simulink model "sampleModel7126_pp_1_1"  (R2018a)
settings: Solver=VariableStepAuto  StartTime=0.0  StopTime=10.0  RelTol=1e-3
undefined symbols (not defined in the file): DiscIntNeverNeededParam
libraries: simulink x367
(part 11 of 12)

== system sampleModel7126_pp_1_1/cfblk298/cfblk16 ==
  cfblk1 : Inport
  Action Port : ActionPort  ActionType=else
  cfblk10 : Subsystem  TreatAsAtomicUnit=on
  cfblk11 : Delay  ShowEnablePort=on
      settings: InputPortMap=u0,e6
  cfblk12 : simulink/Discrete/Transfer Fcn Lead or Lag  PoleZ=0.95  ZeroZ=0.75  ICPrevOutput=0.0  ICPrevInput=0.0  DoSatur=off
      settings: SourceProductName=Simulink  SourceProductBaseCode=SL
  cfblk13 : simulink/Discrete/Transfer Fcn Real Zero  ZeroZ=0.75  ICPrevInput=0.0  DoSatur=off
      settings: SourceProductName=Simulink  SourceProductBaseCode=SL
  cfblk14 : simulink/Continuous/PID Controller (2DOF)  Controller=PID  TimeDomain=Discrete-time  SampleTime=-1  IntegratorMethod=Forward Euler  FilterMethod=Forward Euler  Form=Parallel  UseFilter=on  ControllerParametersSource=internal  P=1  I=1  D=0  N=100  b=1  c=1  InitialConditionSource=internal  InitialConditionForIntegrator=0  InitialConditionForFilter=0  ExternalReset=none  LimitOutput=off  UpperSaturationLimit=inf  LowerSaturationLimit=-inf  LinearizeAsGain=off  AntiWindupMode=none  Kb=1  TrackingMode=off  Kt=1  PParamMin=[]  PParamMax=[]  IParamMin=[]  IParamMax=[]  DParamMin=[]  DParamMax=[]  NParamMin=[]  NParamMax=[]  bParamMin=[]  bParamMax=[]  cParamMin=[]  cParamMax=[]  KbParamMin=[]  KbParamMax=[]  KtParamMin=[]  KtParamMax=[]  POutMin=[]  POutMax=[]  IOutMin=[]  IOutMax=[]  DOutMin=[]  DOutMax=[]  NOutMin=[]  NOutMax=[]  bOutMin=[]  bOutMax=[]  cOutMin=[]  cOutMax=[]  KbOutMin=[]  KbOutMax=[]  KtOutMin=[]  KtOutMax=[]  IntegratorOutMin=[]  IntegratorOutMax=[]  FilterOutMin=[]  FilterOutMax=[]  SumOutMin=[]  SumOutMax=[]  Sum1OutMin=[]  Sum1OutMax=[]  Sum2OutMin=[]  Sum2OutMax=[]  Sum3OutMin=[]  Sum3OutMax=[]  SumI1OutMin=[]  SumI1OutMax=[]  SumI2OutMin=[]  SumI2OutMax=[]  SumI3OutMin=[]  SumI3OutMax=[]  SumDOutMin=[]  SumDOutMax=[]  SaturationOutMin=[]  SaturationOutMax=[]  IntegratorContinuousStateAttributes=''  IntegratorStateMustResolveToSignalObject=off  IntegratorRTWStateStorageClass=Auto  FilterContinuousStateAttributes=''  FilterStateMustResolveToSignalObject=off  FilterRTWStateStorageClass=Auto  DifferentiatorICPrevScaledInput=0  DifferentiatorOutMin=[]  DifferentiatorOutMax=[]  FilterDiffOutCoefMin=[]  FilterDiffOutCoefMax=[]  SumDenOutMin=[]  SumDenOutMax=[]  SumNumOutMin=[]  SumNumOutMax=[]  ReciprocalOutMin=[]  ReciprocalOutMax=[]  DivideOutMin=[]  DivideOutMax=[]  TunerSelectOption=Transfer Function Based (PID Tuner App)
  cfblk15 : Delay
  cfblk16 : Delay
  cfblk3 : DiscreteFir
  cfblk4 : simulink/Discrete/Tapped Delay  vinit=0.0  samptime=-1  NumDelays=1  DelayOrder=Oldest  includeCurrent=off
  cfblk5 : simulink/Discrete/Transfer Fcn Real Zero  ZeroZ=0.75  ICPrevInput=0.0  DoSatur=off
      settings: SourceProductName=Simulink  SourceProductBaseCode=SL
  cfblk6 : Subsystem  TreatAsAtomicUnit=on
  cfblk7 : simulink/Continuous/PID Controller  Controller=PID  TimeDomain=Discrete-time  SampleTime=-1  IntegratorMethod=Forward Euler  FilterMethod=Forward Euler  Form=Parallel  UseFilter=on  ControllerParametersSource=internal  P=1  I=1  D=0  N=100  InitialConditionSource=internal  InitialConditionForIntegrator=0  InitialConditionForFilter=0  ExternalReset=none  LimitOutput=off  UpperSaturationLimit=inf  LowerSaturationLimit=-inf  LinearizeAsGain=off  AntiWindupMode=none  Kb=1  TrackingMode=off  Kt=1  PParamMin=[]  PParamMax=[]  IParamMin=[]  IParamMax=[]  DParamMin=[]  DParamMax=[]  NParamMin=[]  NParamMax=[]  KbParamMin=[]  KbParamMax=[]  KtParamMin=[]  KtParamMax=[]  POutMin=[]  POutMax=[]  IOutMin=[]  IOutMax=[]  DOutMin=[]  DOutMax=[]  NOutMin=[]  NOutMax=[]  KbOutMin=[]  KbOutMax=[]  KtOutMin=[]  KtOutMax=[]  IntegratorOutMin=[]  IntegratorOutMax=[]  FilterOutMin=[]  FilterOutMax=[]  SumOutMin=[]  SumOutMax=[]  SumI1OutMin=[]  SumI1OutMax=[]  SumI2OutMin=[]  SumI2OutMax=[]  SumI3OutMin=[]  SumI3OutMax=[]  SumDOutMin=[]  SumDOutMax=[]  SaturationOutMin=[]  SaturationOutMax=[]  IntegratorContinuousStateAttributes=''  IntegratorStateMustResolveToSignalObject=off  IntegratorRTWStateStorageClass=Auto  FilterContinuousStateAttributes=''  FilterStateMustResolveToSignalObject=off  FilterRTWStateStorageClass=Auto  DifferentiatorICPrevScaledInput=0  DifferentiatorOutMin=[]  DifferentiatorOutMax=[]  FilterDiffOutCoefMin=[]  FilterDiffOutCoefMax=[]  SumDenOutMin=[]  SumDenOutMax=[]  SumNumOutMin=[]  SumNumOutMax=[]  ReciprocalOutMin=[]  ReciprocalOutMax=[]  DivideOutMin=[]  DivideOutMax=[]  TunerSelectOption=Transfer Function Based (PID Tuner App)
  cfblk8 : Subsystem  TreatAsAtomicUnit=on
  cfblk9 : simulink/Discrete/Transfer Fcn Real Zero  ZeroZ=0.75  ICPrevInput=0.0  DoSatur=off
      settings: SourceProductName=Simulink  SourceProductBaseCode=SL
  cyemi_{1315..1330} (16 alike) : DataTypeConversion  OutDataTypeStr=double
  emi_1449 : Subsystem  TreatAsAtomicUnit=on
  emi_1451 : If  IfExpression=0 <= u1  SampleTime=[1 0]
  emi_1452 : DataTypeConversion  OutDataTypeStr=double
  emi_1815 : Subsystem  TreatAsAtomicUnit=on
  emi_1817 : If  IfExpression=0 <= u1
  emi_1818 : DataTypeConversion  OutDataTypeStr=double
  emi_905 : Subsystem  TreatAsAtomicUnit=on
  emi_907 : If  IfExpression=0 <= u1  SampleTime=[1 0]
  emi_908 : DataTypeConversion  OutDataTypeStr=double
  cfblk2 : Outport
  wires:
  cfblk7/1 -> cyemi_1319/1, cyemi_1325/1
  cfblk9/1 -> cyemi_1322/1, cyemi_1326/1
  cfblk1/1 -> cyemi_1315/1
  cyemi_1316/1 -> cfblk11/1
  cfblk15/1 -> cyemi_1316/1
  cyemi_1317/1 -> cfblk11/2
  cfblk14/1 -> cyemi_1317/1
  cyemi_1318/1 -> cfblk12/1
  cyemi_1319/1 -> cfblk13/1
  cyemi_1320/1 -> cfblk14/1
  cfblk12/1 -> cyemi_1320/1
  cyemi_1321/1 -> cfblk14/2
  cfblk16/1 -> cyemi_1321/1
  cyemi_1322/1 -> cfblk15/1
  cyemi_1323/1 -> cfblk16/1
  cyemi_1324/1 -> cfblk3/1
  cfblk13/1 -> cyemi_1324/1
  cyemi_1325/1 -> cfblk4/1
  cyemi_1326/1 -> cfblk5/1
  cfblk3/1 -> cyemi_1327/1
  cyemi_1328/1 -> cfblk7/1
  cfblk5/1 -> cyemi_1328/1
  cfblk4/1 -> cyemi_1329/1, emi_908/1, emi_1818/1
  cyemi_1330/1 -> cfblk9/1
  cfblk11/1 -> cyemi_1330/1
  cyemi_1327/1 -> cfblk6/1(emi_903)
  cfblk6/1(emi_904) -> cyemi_1323/1
  emi_907/1 -> cfblk6/Action
  emi_907/2 -> emi_905/Action
  emi_908/1 -> emi_907/1
  cyemi_1329/1 -> cfblk8/1(emi_1447)
  cfblk8/1(emi_1448) -> cfblk2/1
  emi_1451/1 -> cfblk8/Action
  emi_1451/2 -> emi_1449/Action
  emi_1452/1 -> emi_1451/1
  cyemi_1315/1 -> cfblk10/1(emi_1813)
  cfblk10/1(emi_1814) -> emi_1452/1, cyemi_1318/1
  emi_1817/1 -> cfblk10/Action
  emi_1817/2 -> emi_1815/Action
  emi_1818/1 -> emi_1817/1

== system sampleModel7126_pp_1_1/cfblk298/cfblk3 ==
  emi_1703 : Inport
  Action Port : ActionPort  ActionType=then
  cfblk3 : Delay
  emi_1704 : Outport
  wires:
  emi_1703/1 -> cfblk3/1
  cfblk3/1 -> emi_1704/1

== system sampleModel7126_pp_1_1/cfblk298/cfblk4 ==
  emi_1291 : Inport
  Action Port : ActionPort  ActionType=then
  cfblk4 : Delay
  emi_1292 : Outport
  wires:
  emi_1291/1 -> cfblk4/1
  cfblk4/1 -> emi_1292/1

== system sampleModel7126_pp_1_1/cfblk298/emi_1293 ==
  Action Port : ActionPort  ActionType=else
  emi_1294 : Assertion

== system sampleModel7126_pp_1_1/cfblk298/emi_1705 ==
  Action Port : ActionPort  ActionType=else
  emi_1706 : Assertion

== system sampleModel7126_pp_1_1/cfblk245/cfblk18/cfblk3 ==
  emi_65 : Inport
  Action Port : ActionPort  ActionType=then
  cfblk3 : UnitDelay  SampleTime=-1
  emi_66 : Outport
  wires:
  emi_65/1 -> cfblk3/1
  cfblk3/1 -> emi_66/1

== system sampleModel7126_pp_1_1/cfblk245/cfblk18/cfblk5 ==
  emi_460 : Inport
  Action Port : ActionPort  ActionType=then
  cfblk5 : DiscreteFilter
  emi_461 : Outport
  wires:
  emi_460/1 -> cfblk5/1
  cfblk5/1 -> emi_461/1

== system sampleModel7126_pp_1_1/cfblk245/cfblk18/cfblk7 ==
  emi_202 : Inport
  Action Port : ActionPort  ActionType=then
  cfblk7 : simulink/Discrete/Transfer Fcn Lead or Lag  PoleZ=0.95  ZeroZ=0.75  ICPrevOutput=0.0  ICPrevInput=0.0  DoSatur=off
      settings: SourceProductName=Simulink  SourceProductBaseCode=SL
  emi_203 : Outport
  wires:
  emi_202/1 -> cfblk7/1
  cfblk7/1 -> emi_203/1

== system sampleModel7126_pp_1_1/cfblk245/cfblk18/cfblk8 ==
  emi_1710 : Inport
  emi_1711 : Inport  Port=2
  Action Port : ActionPort  ActionType=then
  cfblk8 : Delay  DelayLengthSource=Input port
      settings: InputPortMap=u0,p1
  emi_1712 : Outport
  wires:
  emi_1710/1 -> cfblk8/1
  emi_1711/1 -> cfblk8/2
  cfblk8/1 -> emi_1712/1

== system sampleModel7126_pp_1_1/cfblk245/cfblk18/emi_1713 ==
  Action Port : ActionPort  ActionType=else
  emi_1714 : Assertion

== system sampleModel7126_pp_1_1/cfblk245/cfblk18/emi_204 ==
  Action Port : ActionPort  ActionType=else
  emi_205 : Assertion

== system sampleModel7126_pp_1_1/cfblk245/cfblk18/emi_462 ==
  Action Port : ActionPort  ActionType=else
  emi_463 : Assertion

== system sampleModel7126_pp_1_1/cfblk245/cfblk18/emi_67 ==
  Action Port : ActionPort  ActionType=else
  emi_68 : Assertion

== system sampleModel7126_pp_1_1/cfblk245/cfblk19/cfblk13 ==
  emi_1942 : Inport
  Action Port : ActionPort  ActionType=then
  cfblk13 : Delay
  emi_1943 : Outport
  wires:
  emi_1942/1 -> cfblk13/1
  cfblk13/1 -> emi_1943/1

== system sampleModel7126_pp_1_1/cfblk245/cfblk19/cfblk6 ==
  emi_2159 : Inport
  Action Port : ActionPort  ActionType=then
  cfblk6 : simulink/Discrete/Transfer Fcn First Order  PoleZ=0.95  ICPrevOutput=0.0  DoSatur=off
      settings: SourceProductName=Simulink
  emi_2160 : Outport
  wires:
  emi_2159/1 -> cfblk6/1
  cfblk6/1 -> emi_2160/1

== system sampleModel7126_pp_1_1/cfblk245/cfblk19/emi_1944 ==
  Action Port : ActionPort  ActionType=else
  emi_1945 : Assertion

== system sampleModel7126_pp_1_1/cfblk245/cfblk19/emi_2161 ==
  Action Port : ActionPort  ActionType=else
  emi_2162 : Assertion

== system sampleModel7126_pp_1_1/cfblk246/cfblk10/cfblk10 ==
  emi_152 : Inport
  Action Port : ActionPort  ActionType=then
  cfblk10 : DiscreteStateSpace  SampleTime=-1
  emi_153 : Outport
  wires:
  emi_152/1 -> cfblk10/1
  cfblk10/1 -> emi_153/1

== system sampleModel7126_pp_1_1/cfblk246/cfblk10/cfblk11 ==
  emi_591 : Inport
  Action Port : ActionPort  ActionType=then
  cfblk11 : simulink/Discrete/Transfer Fcn Lead or Lag  PoleZ=0.95  ZeroZ=0.75  ICPrevOutput=0.0  ICPrevInput=0.0  DoSatur=off
      settings: SourceProductName=Simulink  SourceProductBaseCode=SL
  emi_592 : Outport
  wires:
  emi_591/1 -> cfblk11/1
  cfblk11/1 -> emi_592/1

== system sampleModel7126_pp_1_1/cfblk246/cfblk10/cfblk16 ==
  emi_315 : Inport
  Action Port : ActionPort  ActionType=then
  cfblk16 : Delay
  emi_316 : Outport
  wires:
  emi_315/1 -> cfblk16/1
  cfblk16/1 -> emi_316/1

== system sampleModel7126_pp_1_1/cfblk246/cfblk10/cfblk3 ==
  emi_2130 : Inport
  Action Port : ActionPort  ActionType=then
  cfblk3 : simulink/Discrete/Difference  ICPrevInput=0.0  OutMin=[]  OutMax=[]  OutDataTypeStr=double  OutputDataTypeScalingMode=double  OutDataType=fixdt(1, 16)  OutScaling=2^-10  DoSatur=off
  emi_2131 : Outport
  wires:
  emi_2130/1 -> cfblk3/1
  cfblk3/1 -> emi_2131/1

== system sampleModel7126_pp_1_1/cfblk246/cfblk10/emi_154 ==
  Action Port : ActionPort  ActionType=else
  emi_155 : Assertion

== system sampleModel7126_pp_1_1/cfblk246/cfblk10/emi_2132 ==
  Action Port : ActionPort  ActionType=else
  emi_2133 : Assertion

== system sampleModel7126_pp_1_1/cfblk246/cfblk10/emi_317 ==
  Action Port : ActionPort  ActionType=else
  emi_318 : Assertion

== system sampleModel7126_pp_1_1/cfblk246/cfblk10/emi_593 ==
  Action Port : ActionPort  ActionType=else
  emi_594 : Assertion

== system sampleModel7126_pp_1_1/cfblk246/cfblk9/cfblk7 ==
  emi_1899 : Inport
  Action Port : ActionPort  ActionType=then
  cfblk7 : simulink/Discrete/Transfer Fcn Real Zero  ZeroZ=0.75  ICPrevInput=0.0  DoSatur=off
      settings: SourceProductName=Simulink  SourceProductBaseCode=SL
  emi_1900 : Outport
  wires:
  emi_1899/1 -> cfblk7/1
  cfblk7/1 -> emi_1900/1

== system sampleModel7126_pp_1_1/cfblk246/cfblk9/emi_1901 ==
  Action Port : ActionPort  ActionType=else
  emi_1902 : Assertion

== system sampleModel7126_pp_1_1/cfblk247/cfblk18/cfblk9 ==
  emi_1985 : Inport
  Action Port : ActionPort  ActionType=then
  cfblk9 : simulink/Discrete/Transfer Fcn Real Zero  ZeroZ=0.75  ICPrevInput=0.0  DoSatur=off
      settings: SourceProductName=Simulink  SourceProductBaseCode=SL
  emi_1986 : Outport
  wires:
  emi_1985/1 -> cfblk9/1
  cfblk9/1 -> emi_1986/1

== system sampleModel7126_pp_1_1/cfblk247/cfblk18/emi_1987 ==
  Action Port : ActionPort  ActionType=else
  emi_1988 : Assertion

== system sampleModel7126_pp_1_1/cfblk247/cfblk19/cfblk10 ==
  emi_1024 : Inport
  Action Port : ActionPort  ActionType=then
  cfblk10 : Delay
  emi_1025 : Outport
  wires:
  emi_1024/1 -> cfblk10/1
  cfblk10/1 -> emi_1025/1

== system sampleModel7126_pp_1_1/cfblk247/cfblk19/cfblk14 ==
  emi_280 : Inport
  Action Port : ActionPort  ActionType=then
  cfblk14 : Delay
  emi_281 : Outport
  wires:
  emi_280/1 -> cfblk14/1
  cfblk14/1 -> emi_281/1

== system sampleModel7126_pp_1_1/cfblk247/cfblk19/emi_1026 ==
  Action Port : ActionPort  ActionType=else
  emi_1027 : Assertion

== system sampleModel7126_pp_1_1/cfblk247/cfblk19/emi_282 ==
  Action Port : ActionPort  ActionType=else
  emi_283 : Assertion

== system sampleModel7126_pp_1_1/cfblk252/cfblk15/cfblk14 ==
  emi_2123 : Inport
  Action Port : ActionPort  ActionType=then
  cfblk14 : simulink/Discrete/Transfer Fcn Real Zero  ZeroZ=0.75  ICPrevInput=0.0  DoSatur=off
      settings: SourceProductName=Simulink  SourceProductBaseCode=SL
  emi_2124 : Outport
  wires:
  emi_2123/1 -> cfblk14/1
  cfblk14/1 -> emi_2124/1

== system sampleModel7126_pp_1_1/cfblk252/cfblk15/cfblk3 ==
  emi_690 : Inport
  Action Port : ActionPort  ActionType=then
  cfblk3 : Delay
  emi_691 : Outport
  wires:
  emi_690/1 -> cfblk3/1
  cfblk3/1 -> emi_691/1

== system sampleModel7126_pp_1_1/cfblk252/cfblk15/cfblk4 ==
  emi_2201 : Inport
  emi_2202 : Inport  Port=2
  Action Port : ActionPort  ActionType=then
  cfblk4 : Delay  DelayLengthSource=Input port
      settings: InputPortMap=u0,p1
  emi_2203 : Outport
  wires:
  emi_2201/1 -> cfblk4/1
  emi_2202/1 -> cfblk4/2
  cfblk4/1 -> emi_2203/1

== system sampleModel7126_pp_1_1/cfblk252/cfblk15/cfblk8 ==
  emi_1590 : Inport
  Action Port : ActionPort  ActionType=then
  cfblk8 : simulink/Discrete/Transfer Fcn Real Zero  ZeroZ=0.75  ICPrevInput=0.0  DoSatur=off
      settings: SourceProductName=Simulink  SourceProductBaseCode=SL
  emi_1591 : Outport
  wires:
  emi_1590/1 -> cfblk8/1
  cfblk8/1 -> emi_1591/1

== system sampleModel7126_pp_1_1/cfblk252/cfblk15/emi_1592 ==
  Action Port : ActionPort  ActionType=else
  emi_1593 : Assertion

== system sampleModel7126_pp_1_1/cfblk252/cfblk15/emi_2125 ==
  Action Port : ActionPort  ActionType=else
  emi_2126 : Assertion

== system sampleModel7126_pp_1_1/cfblk252/cfblk15/emi_2204 ==
  Action Port : ActionPort  ActionType=else
  emi_2205 : Assertion

== system sampleModel7126_pp_1_1/cfblk252/cfblk15/emi_692 ==
  Action Port : ActionPort  ActionType=else
  emi_693 : Assertion

== system sampleModel7126_pp_1_1/cfblk252/cfblk16/cfblk13 ==
  emi_259 : Inport
  Action Port : ActionPort  ActionType=then
  cfblk13 : Delay
  emi_260 : Outport
  wires:
  emi_259/1 -> cfblk13/1
  cfblk13/1 -> emi_260/1

== system sampleModel7126_pp_1_1/cfblk252/cfblk16/cfblk3 ==
  emi_109 : Inport
  emi_110 : Inport  Port=2
  Action Port : ActionPort  ActionType=then
  cfblk3 : Delay  DelayLengthSource=Input port
      settings: InputPortMap=u0,p1
  emi_111 : Outport
  wires:
  emi_109/1 -> cfblk3/1
  emi_110/1 -> cfblk3/2
  cfblk3/1 -> emi_111/1

== system sampleModel7126_pp_1_1/cfblk252/cfblk16/cfblk7 ==
  emi_1095 : Inport
  Action Port : ActionPort  ActionType=then
  cfblk7 : DiscreteTransferFcn
  emi_1096 : Outport
  wires:
  emi_1095/1 -> cfblk7/1
  cfblk7/1 -> emi_1096/1

== system sampleModel7126_pp_1_1/cfblk252/cfblk16/emi_1097 ==
  Action Port : ActionPort  ActionType=else
  emi_1098 : Assertion

== system sampleModel7126_pp_1_1/cfblk252/cfblk16/emi_112 ==
  Action Port : ActionPort  ActionType=else
  emi_113 : Assertion

== system sampleModel7126_pp_1_1/cfblk252/cfblk16/emi_261 ==
  Action Port : ActionPort  ActionType=else
  emi_262 : Assertion

== system sampleModel7126_pp_1_1/cfblk253/cfblk10/cfblk11 ==
  emi_2109 : Inport
  Action Port : ActionPort  ActionType=then
  cfblk11 : DiscreteFir
  emi_2110 : Outport
  wires:
  emi_2109/1 -> cfblk11/1
  cfblk11/1 -> emi_2110/1

== system sampleModel7126_pp_1_1/cfblk253/cfblk10/emi_2111 ==
  Action Port : ActionPort  ActionType=else
  emi_2112 : Assertion

== system sampleModel7126_pp_1_1/cfblk256/cfblk11/cfblk3 ==
  emi_1131 : Inport
  Action Port : ActionPort  ActionType=then
  cfblk3 : simulink/Discrete/Tapped Delay  vinit=0.0  samptime=-1  NumDelays=1  DelayOrder=Oldest  includeCurrent=off
  emi_1132 : Outport
  wires:
  emi_1131/1 -> cfblk3/1
  cfblk3/1 -> emi_1132/1

== system sampleModel7126_pp_1_1/cfblk256/cfblk11/cfblk7 ==
  emi_570 : Inport
  Action Port : ActionPort  ActionType=then
  cfblk7 : simulink/Continuous/PID Controller  Controller=PID  TimeDomain=Discrete-time  SampleTime=-1  IntegratorMethod=Forward Euler  FilterMethod=Forward Euler  Form=Parallel  UseFilter=on  ControllerParametersSource=internal  P=1  I=1  D=0  N=100  InitialConditionSource=internal  InitialConditionForIntegrator=0  InitialConditionForFilter=0  ExternalReset=none  LimitOutput=off  UpperSaturationLimit=inf  LowerSaturationLimit=-inf  LinearizeAsGain=off  AntiWindupMode=none  Kb=1  TrackingMode=off  Kt=1  PParamMin=[]  PParamMax=[]  IParamMin=[]  IParamMax=[]  DParamMin=[]  DParamMax=[]  NParamMin=[]  NParamMax=[]  KbParamMin=[]  KbParamMax=[]  KtParamMin=[]  KtParamMax=[]  POutMin=[]  POutMax=[]  IOutMin=[]  IOutMax=[]  DOutMin=[]  DOutMax=[]  NOutMin=[]  NOutMax=[]  KbOutMin=[]  KbOutMax=[]  KtOutMin=[]  KtOutMax=[]  IntegratorOutMin=[]  IntegratorOutMax=[]  FilterOutMin=[]  FilterOutMax=[]  SumOutMin=[]  SumOutMax=[]  SumI1OutMin=[]  SumI1OutMax=[]  SumI2OutMin=[]  SumI2OutMax=[]  SumI3OutMin=[]  SumI3OutMax=[]  SumDOutMin=[]  SumDOutMax=[]  SaturationOutMin=[]  SaturationOutMax=[]  IntegratorContinuousStateAttributes=''  IntegratorStateMustResolveToSignalObject=off  IntegratorRTWStateStorageClass=Auto  FilterContinuousStateAttributes=''  FilterStateMustResolveToSignalObject=off  FilterRTWStateStorageClass=Auto  DifferentiatorICPrevScaledInput=0  DifferentiatorOutMin=[]  DifferentiatorOutMax=[]  FilterDiffOutCoefMin=[]  FilterDiffOutCoefMax=[]  SumDenOutMin=[]  SumDenOutMax=[]  SumNumOutMin=[]  SumNumOutMax=[]  ReciprocalOutMin=[]  ReciprocalOutMax=[]  DivideOutMin=[]  DivideOutMax=[]  TunerSelectOption=Transfer Function Based (PID Tuner App)
  emi_571 : Outport
  wires:
  emi_570/1 -> cfblk7/1
  cfblk7/1 -> emi_571/1

== system sampleModel7126_pp_1_1/cfblk256/cfblk11/emi_1133 ==
  Action Port : ActionPort  ActionType=else
  emi_1134 : Assertion

== system sampleModel7126_pp_1_1/cfblk256/cfblk11/emi_572 ==
  Action Port : ActionPort  ActionType=else
  emi_573 : Assertion

== system sampleModel7126_pp_1_1/cfblk259/cfblk10/cfblk13 ==
  emi_372 : Inport
  Action Port : ActionPort  ActionType=then
  cfblk13 : Delay
  emi_373 : Outport
  wires:
  emi_372/1 -> cfblk13/1
  cfblk13/1 -> emi_373/1

== system sampleModel7126_pp_1_1/cfblk259/cfblk10/cfblk4 ==
  emi_1547 : Inport
  emi_1548 : Inport  Port=2
  Action Port : ActionPort  ActionType=then
  cfblk4 : Delay  ShowEnablePort=on
      settings: InputPortMap=u0,e6
  emi_1549 : Outport
  wires:
  emi_1547/1 -> cfblk4/1
  emi_1548/1 -> cfblk4/2
  cfblk4/1 -> emi_1549/1

== system sampleModel7126_pp_1_1/cfblk259/cfblk10/cfblk6 ==
  emi_811 : Inport
  Action Port : ActionPort  ActionType=then
  cfblk6 : DiscreteTransferFcn
  emi_812 : Outport
  wires:
  emi_811/1 -> cfblk6/1
  cfblk6/1 -> emi_812/1

== system sampleModel7126_pp_1_1/cfblk259/cfblk10/cfblk9 ==
  emi_860 : Inport
  Action Port : ActionPort  ActionType=then
  cfblk9 : DiscreteTransferFcn
  emi_861 : Outport
  wires:
  emi_860/1 -> cfblk9/1
  cfblk9/1 -> emi_861/1

== system sampleModel7126_pp_1_1/cfblk259/cfblk10/emi_1550 ==
  Action Port : ActionPort  ActionType=else
  emi_1551 : Assertion

== system sampleModel7126_pp_1_1/cfblk259/cfblk10/emi_374 ==
  Action Port : ActionPort  ActionType=else
  emi_375 : Assertion

== system sampleModel7126_pp_1_1/cfblk259/cfblk10/emi_813 ==
  Action Port : ActionPort  ActionType=else
  emi_814 : Assertion

== system sampleModel7126_pp_1_1/cfblk259/cfblk10/emi_862 ==
  Action Port : ActionPort  ActionType=else
  emi_863 : Assertion

== system sampleModel7126_pp_1_1/cfblk259/cfblk9/cfblk10 ==
  emi_1145 : Inport
  Action Port : ActionPort  ActionType=then
  cfblk10 : simulink/Discrete/Difference  ICPrevInput=0.0  OutMin=[]  OutMax=[]  OutDataTypeStr=double  OutputDataTypeScalingMode=double  OutDataType=fixdt(1, 16)  OutScaling=2^-10  DoSatur=off
  emi_1146 : Outport
  wires:
  emi_1145/1 -> cfblk10/1
  cfblk10/1 -> emi_1146/1

== system sampleModel7126_pp_1_1/cfblk259/cfblk9/cfblk14 ==
  emi_1892 : Inport
  Action Port : ActionPort  ActionType=then
  cfblk14 : Delay
  emi_1893 : Outport
  wires:
  emi_1892/1 -> cfblk14/1
  cfblk14/1 -> emi_1893/1

== system sampleModel7126_pp_1_1/cfblk259/cfblk9/cfblk8 ==
  emi_400 : Inport
  emi_401 : Inport  Port=2
  Action Port : ActionPort  ActionType=then
  cfblk8 : Delay  DelayLengthSource=Input port
      settings: InputPortMap=u0,p1
  emi_402 : Outport
  wires:
  emi_400/1 -> cfblk8/1
  emi_401/1 -> cfblk8/2
  cfblk8/1 -> emi_402/1

== system sampleModel7126_pp_1_1/cfblk259/cfblk9/cfblk9 ==
  emi_1283 : Inport
  emi_1284 : Inport  Port=2
  Action Port : ActionPort  ActionType=then
  cfblk9 : Delay  DelayLengthSource=Input port
      settings: InputPortMap=u0,p1
  emi_1285 : Outport
  wires:
  emi_1283/1 -> cfblk9/1
  emi_1284/1 -> cfblk9/2
  cfblk9/1 -> emi_1285/1

== system sampleModel7126_pp_1_1/cfblk259/cfblk9/emi_1147 ==
  Action Port : ActionPort  ActionType=else
  emi_1148 : Assertion

== system sampleModel7126_pp_1_1/cfblk259/cfblk9/emi_1286 ==
  Action Port : ActionPort  ActionType=else
  emi_1287 : Assertion

== system sampleModel7126_pp_1_1/cfblk259/cfblk9/emi_1894 ==
  Action Port : ActionPort  ActionType=else
  emi_1895 : Assertion

== system sampleModel7126_pp_1_1/cfblk259/cfblk9/emi_403 ==
  Action Port : ActionPort  ActionType=else
  emi_404 : Assertion

== system sampleModel7126_pp_1_1/cfblk261/cfblk13/cfblk7 ==
  emi_853 : Inport
  Action Port : ActionPort  ActionType=then
  cfblk7 : simulink/Discrete/Transfer Fcn First Order  PoleZ=0.95  ICPrevOutput=0.0  DoSatur=off
      settings: SourceProductName=Simulink
  emi_854 : Outport
  wires:
  emi_853/1 -> cfblk7/1
  cfblk7/1 -> emi_854/1

== system sampleModel7126_pp_1_1/cfblk261/cfblk13/emi_855 ==
  Action Port : ActionPort  ActionType=else
  emi_856 : Assertion

== system sampleModel7126_pp_1_1/cfblk263/cfblk15/cfblk10 ==
  emi_739 : Inport
  Action Port : ActionPort  ActionType=then
  cfblk10 : DiscreteZeroPole  Poles=[0 0.5]  Gain=1  SampleTime=-1
  emi_740 : Outport
  wires:
  emi_739/1 -> cfblk10/1
  cfblk10/1 -> emi_740/1

== system sampleModel7126_pp_1_1/cfblk263/cfblk15/cfblk3 ==
  emi_917 : Inport
  Action Port : ActionPort  ActionType=then
  cfblk3 : simulink/Discrete/Difference  ICPrevInput=0.0  OutMin=[]  OutMax=[]  OutDataTypeStr=fixdt('ufix32_En8')  OutputDataTypeScalingMode=Specify via dialog  OutDataType=fixdt('ufix32_En8')  OutScaling=[]  DoSatur=off
  emi_918 : Outport
  wires:
  emi_917/1 -> cfblk3/1
  cfblk3/1 -> emi_918/1

== system sampleModel7126_pp_1_1/cfblk263/cfblk15/cfblk8 ==
  emi_781 : Inport
  emi_782 : Inport  Port=2
  Action Port : ActionPort  ActionType=then
  cfblk8 : simulink/Continuous/PID Controller (2DOF)  Controller=PID  TimeDomain=Discrete-time  SampleTime=-1  IntegratorMethod=Forward Euler  FilterMethod=Forward Euler  Form=Parallel  UseFilter=on  ControllerParametersSource=internal  P=1  I=1  D=0  N=100  b=1  c=1  InitialConditionSource=internal  InitialConditionForIntegrator=0  InitialConditionForFilter=0  ExternalReset=none  LimitOutput=off  UpperSaturationLimit=inf  LowerSaturationLimit=-inf  LinearizeAsGain=off  AntiWindupMode=none  Kb=1  TrackingMode=off  Kt=1  PParamMin=[]  PParamMax=[]  IParamMin=[]  IParamMax=[]  DParamMin=[]  DParamMax=[]  NParamMin=[]  NParamMax=[]  bParamMin=[]  bParamMax=[]  cParamMin=[]  cParamMax=[]  KbParamMin=[]  KbParamMax=[]  KtParamMin=[]  KtParamMax=[]  POutMin=[]  POutMax=[]  IOutMin=[]  IOutMax=[]  DOutMin=[]  DOutMax=[]  NOutMin=[]  NOutMax=[]  bOutMin=[]  bOutMax=[]  cOutMin=[]  cOutMax=[]  KbOutMin=[]  KbOutMax=[]  KtOutMin=[]  KtOutMax=[]  IntegratorOutMin=[]  IntegratorOutMax=[]  FilterOutMin=[]  FilterOutMax=[]  SumOutMin=[]  SumOutMax=[]  Sum1OutMin=[]  Sum1OutMax=[]  Sum2OutMin=[]  Sum2OutMax=[]  Sum3OutMin=[]  Sum3OutMax=[]  SumI1OutMin=[]  SumI1OutMax=[]  SumI2OutMin=[]  SumI2OutMax=[]  SumI3OutMin=[]  SumI3OutMax=[]  SumDOutMin=[]  SumDOutMax=[]  SaturationOutMin=[]  SaturationOutMax=[]  IntegratorContinuousStateAttributes=''  IntegratorStateMustResolveToSignalObject=off  IntegratorRTWStateStorageClass=Auto  FilterContinuousStateAttributes=''  FilterStateMustResolveToSignalObject=off  FilterRTWStateStorageClass=Auto  DifferentiatorICPrevScaledInput=0  DifferentiatorOutMin=[]  DifferentiatorOutMax=[]  FilterDiffOutCoefMin=[]  FilterDiffOutCoefMax=[]  SumDenOutMin=[]  SumDenOutMax=[]  SumNumOutMin=[]  SumNumOutMax=[]  ReciprocalOutMin=[]  ReciprocalOutMax=[]  DivideOutMin=[]  DivideOutMax=[]  TunerSelectOption=Transfer Function Based (PID Tuner App)
  emi_783 : Outport
  wires:
  emi_781/1 -> cfblk8/1
  emi_782/1 -> cfblk8/2
  cfblk8/1 -> emi_783/1

== system sampleModel7126_pp_1_1/cfblk263/cfblk15/emi_741 ==
  Action Port : ActionPort  ActionType=else
  emi_742 : Assertion

== system sampleModel7126_pp_1_1/cfblk263/cfblk15/emi_784 ==
  Action Port : ActionPort  ActionType=else
  emi_785 : Assertion

== system sampleModel7126_pp_1_1/cfblk263/cfblk15/emi_919 ==
  Action Port : ActionPort  ActionType=else
  emi_920 : Assertion

== system sampleModel7126_pp_1_1/cfblk263/cfblk16/cfblk3 ==
  emi_1978 : Inport
  Action Port : ActionPort  ActionType=then
  cfblk3 : DiscreteFir
  emi_1979 : Outport
  wires:
  emi_1978/1 -> cfblk3/1
  cfblk3/1 -> emi_1979/1

== system sampleModel7126_pp_1_1/cfblk263/cfblk16/cfblk4 ==
  emi_1555 : Inport
  Action Port : ActionPort  ActionType=then
  cfblk4 : simulink/Discrete/Tapped Delay  vinit=0.0  samptime=-1  NumDelays=1  DelayOrder=Oldest  includeCurrent=off
  emi_1556 : Outport
  wires:
  emi_1555/1 -> cfblk4/1
  cfblk4/1 -> emi_1556/1

== system sampleModel7126_pp_1_1/cfblk263/cfblk16/cfblk5 ==
  emi_676 : Inport
  Action Port : ActionPort  ActionType=then
  cfblk5 : simulink/Discrete/Transfer Fcn Real Zero  ZeroZ=0.75  ICPrevInput=0.0  DoSatur=off
      settings: SourceProductName=Simulink  SourceProductBaseCode=SL
  emi_677 : Outport
  wires:
  emi_676/1 -> cfblk5/1
  cfblk5/1 -> emi_677/1

== system sampleModel7126_pp_1_1/cfblk263/cfblk16/cfblk6 ==
  emi_910 : Inport
  Action Port : ActionPort  ActionType=then
  cfblk6 : UnitDelay  SampleTime=-1
  emi_911 : Outport
  wires:
  emi_910/1 -> cfblk6/1
  cfblk6/1 -> emi_911/1

== system sampleModel7126_pp_1_1/cfblk263/cfblk16/emi_1557 ==
  Action Port : ActionPort  ActionType=else
  emi_1558 : Assertion

== system sampleModel7126_pp_1_1/cfblk263/cfblk16/emi_1980 ==
  Action Port : ActionPort  ActionType=else
  emi_1981 : Assertion

== system sampleModel7126_pp_1_1/cfblk263/cfblk16/emi_678 ==
  Action Port : ActionPort  ActionType=else
  emi_679 : Assertion

== system sampleModel7126_pp_1_1/cfblk263/cfblk16/emi_912 ==
  Action Port : ActionPort  ActionType=else
  emi_913 : Assertion

== system sampleModel7126_pp_1_1/cfblk265/cfblk10/cfblk6 ==
  emi_931 : Inport
  Action Port : ActionPort  ActionType=then
  cfblk6 : simulink/Discrete/Difference  ICPrevInput=0.0  OutMin=[]  OutMax=[]  OutDataTypeStr=double  OutputDataTypeScalingMode=double  OutDataType=fixdt(1, 16)  OutScaling=2^-10  DoSatur=off
  emi_932 : Outport
  wires:
  emi_931/1 -> cfblk6/1
  cfblk6/1 -> emi_932/1

== system sampleModel7126_pp_1_1/cfblk265/cfblk10/emi_933 ==
  Action Port : ActionPort  ActionType=else
  emi_934 : Assertion

== system sampleModel7126_pp_1_1/cfblk266/cfblk10/cfblk3 ==
  emi_266 : Inport
  Action Port : ActionPort  ActionType=then
  cfblk3 : DiscreteZeroPole  Poles=[0 0.5]  Gain=1  SampleTime=-1
  emi_267 : Outport
  wires:
  emi_266/1 -> cfblk3/1
  cfblk3/1 -> emi_267/1

== system sampleModel7126_pp_1_1/cfblk266/cfblk10/cfblk4 ==
  emi_1877 : Inport
  emi_1878 : Inport  Port=2
  Action Port : ActionPort  ActionType=then
  cfblk4 : simulink/Continuous/PID Controller (2DOF)  Controller=PID  TimeDomain=Discrete-time  SampleTime=-1  IntegratorMethod=Forward Euler  FilterMethod=Forward Euler  Form=Parallel  UseFilter=on  ControllerParametersSource=internal  P=1  I=1  D=0  N=100  b=1  c=1  InitialConditionSource=internal  InitialConditionForIntegrator=0  InitialConditionForFilter=0  ExternalReset=none  LimitOutput=off  UpperSaturationLimit=inf  LowerSaturationLimit=-inf  LinearizeAsGain=off  AntiWindupMode=none  Kb=1  TrackingMode=off  Kt=1  PParamMin=[]  PParamMax=[]  IParamMin=[]  IParamMax=[]  DParamMin=[]  DParamMax=[]  NParamMin=[]  NParamMax=[]  bParamMin=[]  bParamMax=[]  cParamMin=[]  cParamMax=[]  KbParamMin=[]  KbParamMax=[]  KtParamMin=[]  KtParamMax=[]  POutMin=[]  POutMax=[]  IOutMin=[]  IOutMax=[]  DOutMin=[]  DOutMax=[]  NOutMin=[]  NOutMax=[]  bOutMin=[]  bOutMax=[]  cOutMin=[]  cOutMax=[]  KbOutMin=[]  KbOutMax=[]  KtOutMin=[]  KtOutMax=[]  IntegratorOutMin=[]  IntegratorOutMax=[]  FilterOutMin=[]  FilterOutMax=[]  SumOutMin=[]  SumOutMax=[]  Sum1OutMin=[]  Sum1OutMax=[]  Sum2OutMin=[]  Sum2OutMax=[]  Sum3OutMin=[]  Sum3OutMax=[]  SumI1OutMin=[]  SumI1OutMax=[]  SumI2OutMin=[]  SumI2OutMax=[]  SumI3OutMin=[]  SumI3OutMax=[]  SumDOutMin=[]  SumDOutMax=[]  SaturationOutMin=[]  SaturationOutMax=[]  IntegratorContinuousStateAttributes=''  IntegratorStateMustResolveToSignalObject=off  IntegratorRTWStateStorageClass=Auto  FilterContinuousStateAttributes=''  FilterStateMustResolveToSignalObject=off  FilterRTWStateStorageClass=Auto  DifferentiatorICPrevScaledInput=0  DifferentiatorOutMin=[]  DifferentiatorOutMax=[]  FilterDiffOutCoefMin=[]  FilterDiffOutCoefMax=[]  SumDenOutMin=[]  SumDenOutMax=[]  SumNumOutMin=[]  SumNumOutMax=[]  ReciprocalOutMin=[]  ReciprocalOutMax=[]  DivideOutMin=[]  DivideOutMax=[]  TunerSelectOption=Transfer Function Based (PID Tuner App)
  emi_1879 : Outport
  wires:
  emi_1877/1 -> cfblk4/1
  emi_1878/1 -> cfblk4/2
  cfblk4/1 -> emi_1879/1

== system sampleModel7126_pp_1_1/cfblk266/cfblk10/cfblk5 ==
  emi_520 : Inport
  emi_521 : Inport  Port=2
  Action Port : ActionPort  ActionType=then
  cfblk5 : Delay  ShowEnablePort=on
      settings: InputPortMap=u0,e6
  emi_522 : Outport
  wires:
  emi_520/1 -> cfblk5/1
  emi_521/1 -> cfblk5/2
  cfblk5/1 -> emi_522/1

== system sampleModel7126_pp_1_1/cfblk266/cfblk10/cfblk8 ==
  emi_612 : Inport
  Action Port : ActionPort  ActionType=then
  cfblk8 : Delay
  emi_613 : Outport
  wires:
  emi_612/1 -> cfblk8/1
  cfblk8/1 -> emi_613/1

== system sampleModel7126_pp_1_1/cfblk266/cfblk10/emi_1880 ==
  Action Port : ActionPort  ActionType=else
  emi_1881 : Assertion

== system sampleModel7126_pp_1_1/cfblk266/cfblk10/emi_268 ==
  Action Port : ActionPort  ActionType=else
  emi_269 : Assertion

== system sampleModel7126_pp_1_1/cfblk266/cfblk10/emi_523 ==
  Action Port : ActionPort  ActionType=else
  emi_524 : Assertion

== system sampleModel7126_pp_1_1/cfblk266/cfblk10/emi_614 ==
  Action Port : ActionPort  ActionType=else
  emi_615 : Assertion

== system sampleModel7126_pp_1_1/cfblk269/cfblk8/cfblk11 ==
  emi_953 : Inport
  Action Port : ActionPort  ActionType=then
  cfblk11 : DiscreteStateSpace  SampleTime=-1
  emi_954 : Outport
  wires:
  emi_953/1 -> cfblk11/1
  cfblk11/1 -> emi_954/1

== system sampleModel7126_pp_1_1/cfblk269/cfblk8/cfblk7 ==
  emi_2073 : Inport
  Action Port : ActionPort  ActionType=then
  cfblk7 : DiscreteStateSpace  SampleTime=-1
  emi_2074 : Outport
  wires:
  emi_2073/1 -> cfblk7/1
  cfblk7/1 -> emi_2074/1

== system sampleModel7126_pp_1_1/cfblk269/cfblk8/emi_2075 ==
  Action Port : ActionPort  ActionType=else
  emi_2076 : Assertion

== system sampleModel7126_pp_1_1/cfblk269/cfblk8/emi_955 ==
  Action Port : ActionPort  ActionType=else
  emi_956 : Assertion

== system sampleModel7126_pp_1_1/cfblk269/cfblk9/cfblk5 ==
  emi_1195 : Inport
  emi_1196 : Inport  Port=2
  Action Port : ActionPort  ActionType=then
  cfblk5 : Delay  ShowEnablePort=on
      settings: InputPortMap=u0,e6
  emi_1197 : Outport
  wires:
  emi_1195/1 -> cfblk5/1
  emi_1196/1 -> cfblk5/2
  cfblk5/1 -> emi_1197/1

== system sampleModel7126_pp_1_1/cfblk269/cfblk9/cfblk6 ==
  emi_273 : Inport
  Action Port : ActionPort  ActionType=then
  cfblk6 : simulink/Discrete/Tapped Delay  vinit=0.0  samptime=-1  NumDelays=1  DelayOrder=Oldest  includeCurrent=off
  emi_274 : Outport
  wires:
  emi_273/1 -> cfblk6/1
  cfblk6/1 -> emi_274/1

== system sampleModel7126_pp_1_1/cfblk269/cfblk9/emi_1198 ==
  Action Port : ActionPort  ActionType=else
  emi_1199 : Assertion

== system sampleModel7126_pp_1_1/cfblk269/cfblk9/emi_275 ==
  Action Port : ActionPort  ActionType=else
  emi_276 : Assertion

== system sampleModel7126_pp_1_1/cfblk273/cfblk10/cfblk3 ==
  emi_180 : Inport
  Action Port : ActionPort  ActionType=then
  cfblk3 : DiscreteStateSpace  SampleTime=-1
  emi_181 : Outport
  wires:
  emi_180/1 -> cfblk3/1
  cfblk3/1 -> emi_181/1

== system sampleModel7126_pp_1_1/cfblk273/cfblk10/cfblk4 ==
  emi_1518 : Inport
  Action Port : ActionPort  ActionType=then
  cfblk4 : DiscreteStateSpace  SampleTime=-1
  emi_1519 : Outport
  wires:
  emi_1518/1 -> cfblk4/1
  cfblk4/1 -> emi_1519/1

== system sampleModel7126_pp_1_1/cfblk273/cfblk10/cfblk5 ==
  emi_1074 : Inport
  Action Port : ActionPort  ActionType=then
  cfblk5 : DiscreteTransferFcn
  emi_1075 : Outport
  wires:
  emi_1074/1 -> cfblk5/1
  cfblk5/1 -> emi_1075/1

== system sampleModel7126_pp_1_1/cfblk273/cfblk10/emi_1076 ==
  Action Port : ActionPort  ActionType=else
  emi_1077 : Assertion

== system sampleModel7126_pp_1_1/cfblk273/cfblk10/emi_1520 ==
  Action Port : ActionPort  ActionType=else
  emi_1521 : Assertion

== system sampleModel7126_pp_1_1/cfblk273/cfblk10/emi_182 ==
  Action Port : ActionPort  ActionType=else
  emi_183 : Assertion

== system sampleModel7126_pp_1_1/cfblk273/cfblk9/cfblk16 ==
  emi_1957 : Inport
  Action Port : ActionPort  ActionType=then
  cfblk16 : Delay
  emi_1958 : Outport
  wires:
  emi_1957/1 -> cfblk16/1
  cfblk16/1 -> emi_1958/1

== system sampleModel7126_pp_1_1/cfblk273/cfblk9/cfblk3 ==
  emi_1369 : Inport
  Action Port : ActionPort  ActionType=then
  cfblk3 : UnitDelay  SampleTime=-1
  emi_1370 : Outport
  wires:
  emi_1369/1 -> cfblk3/1
  cfblk3/1 -> emi_1370/1

== system sampleModel7126_pp_1_1/cfblk273/cfblk9/cfblk5 ==
  emi_1002 : Inport
  emi_1003 : Inport  Port=2
  Action Port : ActionPort  ActionType=then
  cfblk5 : Delay  ShowEnablePort=on
      settings: InputPortMap=u0,e6
  emi_1004 : Outport
  wires:
  emi_1002/1 -> cfblk5/1
  emi_1003/1 -> cfblk5/2
  cfblk5/1 -> emi_1004/1

== system sampleModel7126_pp_1_1/cfblk273/cfblk9/cfblk8 ==
  emi_874 : Inport
  Action Port : ActionPort  ActionType=then
  cfblk8 : DiscreteIntegrator  SampleTime=-1  OutDataTypeStr=double  ICPrevOutput=DiscIntNeverNeededParam  ICPrevScaledInput=DiscIntNeverNeededParam
  emi_875 : Outport
  wires:
  emi_874/1 -> cfblk8/1
  cfblk8/1 -> emi_875/1

== system sampleModel7126_pp_1_1/cfblk273/cfblk9/emi_1005 ==
  Action Port : ActionPort  ActionType=else
  emi_1006 : Assertion

== system sampleModel7126_pp_1_1/cfblk273/cfblk9/emi_1371 ==
  Action Port : ActionPort  ActionType=else
  emi_1372 : Assertion

== system sampleModel7126_pp_1_1/cfblk273/cfblk9/emi_1959 ==
  Action Port : ActionPort  ActionType=else
  emi_1960 : Assertion

== system sampleModel7126_pp_1_1/cfblk273/cfblk9/emi_876 ==
  Action Port : ActionPort  ActionType=else
  emi_877 : Assertion

== system sampleModel7126_pp_1_1/cfblk275/cfblk10/cfblk3 ==
  emi_1696 : Inport
  Action Port : ActionPort  ActionType=then
  cfblk3 : DiscreteFir
  emi_1697 : Outport
  wires:
  emi_1696/1 -> cfblk3/1
  cfblk3/1 -> emi_1697/1

== system sampleModel7126_pp_1_1/cfblk275/cfblk10/cfblk4 ==
  emi_1935 : Inport
  Action Port : ActionPort  ActionType=then
  cfblk4 : simulink/Discrete/Transfer Fcn Lead or Lag  PoleZ=0.95  ZeroZ=0.75  ICPrevOutput=0.0  ICPrevInput=0.0  DoSatur=off
      settings: SourceProductName=Simulink  SourceProductBaseCode=SL
  emi_1936 : Outport
  wires:
  emi_1935/1 -> cfblk4/1
  cfblk4/1 -> emi_1936/1

== system sampleModel7126_pp_1_1/cfblk275/cfblk10/cfblk5 ==
  emi_124 : Inport
  Action Port : ActionPort  ActionType=then
  cfblk5 : simulink/Discrete/Transfer Fcn Lead or Lag  PoleZ=0.95  ZeroZ=0.75  ICPrevOutput=0.0  ICPrevInput=0.0  DoSatur=off
      settings: SourceProductName=Simulink  SourceProductBaseCode=SL
  emi_125 : Outport
  wires:
  emi_124/1 -> cfblk5/1
  cfblk5/1 -> emi_125/1

== system sampleModel7126_pp_1_1/cfblk275/cfblk10/cfblk8 ==
  emi_1203 : Inport
  Action Port : ActionPort  ActionType=then
  cfblk8 : DiscreteTransferFcn
  emi_1204 : Outport
  wires:
  emi_1203/1 -> cfblk8/1
  cfblk8/1 -> emi_1204/1

== system sampleModel7126_pp_1_1/cfblk275/cfblk10/emi_1205 ==
  Action Port : ActionPort  ActionType=else
  emi_1206 : Assertion

== system sampleModel7126_pp_1_1/cfblk275/cfblk10/emi_126 ==
  Action Port : ActionPort  ActionType=else
  emi_127 : Assertion

== system sampleModel7126_pp_1_1/cfblk275/cfblk10/emi_1698 ==
  Action Port : ActionPort  ActionType=else
  emi_1699 : Assertion

== system sampleModel7126_pp_1_1/cfblk275/cfblk10/emi_1937 ==
  Action Port : ActionPort  ActionType=else
  emi_1938 : Assertion

== system sampleModel7126_pp_1_1/cfblk275/cfblk11/cfblk11 ==
  emi_2187 : Inport
  Action Port : ActionPort  ActionType=then
  cfblk11 : DiscreteFilter
  emi_2188 : Outport
  wires:
  emi_2187/1 -> cfblk11/1
  cfblk11/1 -> emi_2188/1

== system sampleModel7126_pp_1_1/cfblk275/cfblk11/cfblk14 ==
  emi_563 : Inport
  Action Port : ActionPort  ActionType=then
  cfblk14 : DiscreteFilter
  emi_564 : Outport
  wires:
  emi_563/1 -> cfblk14/1
  cfblk14/1 -> emi_564/1

== system sampleModel7126_pp_1_1/cfblk275/cfblk11/cfblk3 ==
  emi_605 : Inport
  Action Port : ActionPort  ActionType=then
  cfblk3 : DiscreteStateSpace  SampleTime=-1
  emi_606 : Outport
  wires:
  emi_605/1 -> cfblk3/1
  cfblk3/1 -> emi_606/1

== system sampleModel7126_pp_1_1/cfblk275/cfblk11/cfblk9 ==
  emi_1320 : Inport
  Action Port : ActionPort  ActionType=then
  cfblk9 : DiscreteFilter
  emi_1321 : Outport
  wires:
  emi_1320/1 -> cfblk9/1
  cfblk9/1 -> emi_1321/1

== system sampleModel7126_pp_1_1/cfblk275/cfblk11/emi_1322 ==
  Action Port : ActionPort  ActionType=else
  emi_1323 : Assertion

== system sampleModel7126_pp_1_1/cfblk275/cfblk11/emi_2189 ==
  Action Port : ActionPort  ActionType=else
  emi_2190 : Assertion

== system sampleModel7126_pp_1_1/cfblk275/cfblk11/emi_565 ==
  Action Port : ActionPort  ActionType=else
  emi_566 : Assertion

== system sampleModel7126_pp_1_1/cfblk275/cfblk11/emi_607 ==
  Action Port : ActionPort  ActionType=else
  emi_608 : Assertion

== system sampleModel7126_pp_1_1/cfblk277/cfblk18/cfblk3 ==
  emi_549 : Inport
  Action Port : ActionPort  ActionType=then
  cfblk3 : simulink/Discrete/Transfer Fcn Real Zero  ZeroZ=0.75  ICPrevInput=0.0  DoSatur=off
      settings: SourceProductName=Simulink  SourceProductBaseCode=SL
  emi_550 : Outport
  wires:
  emi_549/1 -> cfblk3/1
  cfblk3/1 -> emi_550/1

== system sampleModel7126_pp_1_1/cfblk277/cfblk18/cfblk5 ==
  emi_938 : Inport
  Action Port : ActionPort  ActionType=then
  cfblk5 : DiscreteIntegrator  SampleTime=-1  OutDataTypeStr=double  ICPrevOutput=DiscIntNeverNeededParam  ICPrevScaledInput=DiscIntNeverNeededParam
  emi_939 : Outport
  wires:
  emi_938/1 -> cfblk5/1
  cfblk5/1 -> emi_939/1

== system sampleModel7126_pp_1_1/cfblk277/cfblk18/cfblk7 ==
  emi_2151 : Inport
  emi_2152 : Inport  Port=2
  Action Port : ActionPort  ActionType=then
  cfblk7 : simulink/Continuous/PID Controller (2DOF)  Controller=PID  TimeDomain=Discrete-time  SampleTime=-1  IntegratorMethod=Forward Euler  FilterMethod=Forward Euler  Form=Parallel  UseFilter=on  ControllerParametersSource=internal  P=1  I=1  D=0  N=100  b=1  c=1  InitialConditionSource=internal  InitialConditionForIntegrator=0  InitialConditionForFilter=0  ExternalReset=none  LimitOutput=off  UpperSaturationLimit=inf  LowerSaturationLimit=-inf  LinearizeAsGain=off  AntiWindupMode=none  Kb=1  TrackingMode=off  Kt=1  PParamMin=[]  PParamMax=[]  IParamMin=[]  IParamMax=[]  DParamMin=[]  DParamMax=[]  NParamMin=[]  NParamMax=[]  bParamMin=[]  bParamMax=[]  cParamMin=[]  cParamMax=[]  KbParamMin=[]  KbParamMax=[]  KtParamMin=[]  KtParamMax=[]  POutMin=[]  POutMax=[]  IOutMin=[]  IOutMax=[]  DOutMin=[]  DOutMax=[]  NOutMin=[]  NOutMax=[]  bOutMin=[]  bOutMax=[]  cOutMin=[]  cOutMax=[]  KbOutMin=[]  KbOutMax=[]  KtOutMin=[]  KtOutMax=[]  IntegratorOutMin=[]  IntegratorOutMax=[]  FilterOutMin=[]  FilterOutMax=[]  SumOutMin=[]  SumOutMax=[]  Sum1OutMin=[]  Sum1OutMax=[]  Sum2OutMin=[]  Sum2OutMax=[]  Sum3OutMin=[]  Sum3OutMax=[]  SumI1OutMin=[]  SumI1OutMax=[]  SumI2OutMin=[]  SumI2OutMax=[]  SumI3OutMin=[]  SumI3OutMax=[]  SumDOutMin=[]  SumDOutMax=[]  SaturationOutMin=[]  SaturationOutMax=[]  IntegratorContinuousStateAttributes=''  IntegratorStateMustResolveToSignalObject=off  IntegratorRTWStateStorageClass=Auto  FilterContinuousStateAttributes=''  FilterStateMustResolveToSignalObject=off  FilterRTWStateStorageClass=Auto  DifferentiatorICPrevScaledInput=0  DifferentiatorOutMin=[]  DifferentiatorOutMax=[]  FilterDiffOutCoefMin=[]  FilterDiffOutCoefMax=[]  SumDenOutMin=[]  SumDenOutMax=[]  SumNumOutMin=[]  SumNumOutMax=[]  ReciprocalOutMin=[]  ReciprocalOutMax=[]  DivideOutMin=[]  DivideOutMax=[]  TunerSelectOption=Transfer Function Based (PID Tuner App)
  emi_2153 : Outport
  wires:
  emi_2151/1 -> cfblk7/1
  emi_2152/1 -> cfblk7/2
  cfblk7/1 -> emi_2153/1

== system sampleModel7126_pp_1_1/cfblk277/cfblk18/emi_2154 ==
  Action Port : ActionPort  ActionType=else
  emi_2155 : Assertion

== system sampleModel7126_pp_1_1/cfblk277/cfblk18/emi_551 ==
  Action Port : ActionPort  ActionType=else
  emi_552 : Assertion

== system sampleModel7126_pp_1_1/cfblk277/cfblk18/emi_940 ==
  Action Port : ActionPort  ActionType=else
  emi_941 : Assertion

== system sampleModel7126_pp_1_1/cfblk277/cfblk19/cfblk5 ==
  emi_1906 : Inport
  Action Port : ActionPort  ActionType=then
  cfblk5 : DiscreteIntegrator  SampleTime=-1  OutDataTypeStr=double  ICPrevOutput=DiscIntNeverNeededParam  ICPrevScaledInput=DiscIntNeverNeededParam
  emi_1907 : Outport
  wires:
  emi_1906/1 -> cfblk5/1
  cfblk5/1 -> emi_1907/1

== system sampleModel7126_pp_1_1/cfblk277/cfblk19/cfblk6 ==
  emi_379 : Inport
  Action Port : ActionPort  ActionType=then
  cfblk6 : DiscreteFilter
  emi_380 : Outport
  wires:
  emi_379/1 -> cfblk6/1
  cfblk6/1 -> emi_380/1

== system sampleModel7126_pp_1_1/cfblk277/cfblk19/cfblk8 ==
  emi_1597 : Inport
  Action Port : ActionPort  ActionType=then
  cfblk8 : simulink/Continuous/PID Controller  Controller=PID  TimeDomain=Discrete-time  SampleTime=-1  IntegratorMethod=Forward Euler  FilterMethod=Forward Euler  Form=Parallel  UseFilter=on  ControllerParametersSource=internal  P=1  I=1  D=0  N=100  InitialConditionSource=internal  InitialConditionForIntegrator=0  InitialConditionForFilter=0  ExternalReset=none  LimitOutput=off  UpperSaturationLimit=inf  LowerSaturationLimit=-inf  LinearizeAsGain=off  AntiWindupMode=none  Kb=1  TrackingMode=off  Kt=1  PParamMin=[]  PParamMax=[]  IParamMin=[]  IParamMax=[]  DParamMin=[]  DParamMax=[]  NParamMin=[]  NParamMax=[]  KbParamMin=[]  KbParamMax=[]  KtParamMin=[]  KtParamMax=[]  POutMin=[]  POutMax=[]  IOutMin=[]  IOutMax=[]  DOutMin=[]  DOutMax=[]  NOutMin=[]  NOutMax=[]  KbOutMin=[]  KbOutMax=[]  KtOutMin=[]  KtOutMax=[]  IntegratorOutMin=[]  IntegratorOutMax=[]  FilterOutMin=[]  FilterOutMax=[]  SumOutMin=[]  SumOutMax=[]  SumI1OutMin=[]  SumI1OutMax=[]  SumI2OutMin=[]  SumI2OutMax=[]  SumI3OutMin=[]  SumI3OutMax=[]  SumDOutMin=[]  SumDOutMax=[]  SaturationOutMin=[]  SaturationOutMax=[]  IntegratorContinuousStateAttributes=''  IntegratorStateMustResolveToSignalObject=off  IntegratorRTWStateStorageClass=Auto  FilterContinuousStateAttributes=''  FilterStateMustResolveToSignalObject=off  FilterRTWStateStorageClass=Auto  DifferentiatorICPrevScaledInput=0  DifferentiatorOutMin=[]  DifferentiatorOutMax=[]  FilterDiffOutCoefMin=[]  FilterDiffOutCoefMax=[]  SumDenOutMin=[]  SumDenOutMax=[]  SumNumOutMin=[]  SumNumOutMax=[]  ReciprocalOutMin=[]  ReciprocalOutMax=[]  DivideOutMin=[]  DivideOutMax=[]  TunerSelectOption=Transfer Function Based (PID Tuner App)
  emi_1598 : Outport
  wires:
  emi_1597/1 -> cfblk8/1
  cfblk8/1 -> emi_1598/1

== system sampleModel7126_pp_1_1/cfblk277/cfblk19/emi_1599 ==
  Action Port : ActionPort  ActionType=else
  emi_1600 : Assertion

== system sampleModel7126_pp_1_1/cfblk277/cfblk19/emi_1908 ==
  Action Port : ActionPort  ActionType=else
  emi_1909 : Assertion

== system sampleModel7126_pp_1_1/cfblk277/cfblk19/emi_381 ==
  Action Port : ActionPort  ActionType=else
  emi_382 : Assertion

== system sampleModel7126_pp_1_1/cfblk278/cfblk12/cfblk12 ==
  emi_2137 : Inport
  Action Port : ActionPort  ActionType=then
  cfblk12 : DiscreteTransferFcn
  emi_2138 : Outport
  wires:
  emi_2137/1 -> cfblk12/1
  cfblk12/1 -> emi_2138/1

== system sampleModel7126_pp_1_1/cfblk278/cfblk12/cfblk6 ==
  emi_72 : Inport
  Action Port : ActionPort  ActionType=then
  cfblk6 : DiscreteStateSpace  SampleTime=-1
  emi_73 : Outport
  wires:
  emi_72/1 -> cfblk6/1
  cfblk6/1 -> emi_73/1

== system sampleModel7126_pp_1_1/cfblk278/cfblk12/emi_2139 ==
  Action Port : ActionPort  ActionType=else
  emi_2140 : Assertion

== system sampleModel7126_pp_1_1/cfblk278/cfblk12/emi_74 ==
  Action Port : ActionPort  ActionType=else
  emi_75 : Assertion

== system sampleModel7126_pp_1_1/cfblk278/cfblk15/cfblk4 ==
  emi_655 : Inport
  Action Port : ActionPort  ActionType=then
  cfblk4 : simulink/Continuous/PID Controller  Controller=PID  TimeDomain=Discrete-time  SampleTime=-1  IntegratorMethod=Forward Euler  FilterMethod=Forward Euler  Form=Parallel  UseFilter=on  ControllerParametersSource=internal  P=1  I=1  D=0  N=100  InitialConditionSource=internal  InitialConditionForIntegrator=0  InitialConditionForFilter=0  ExternalReset=none  LimitOutput=off  UpperSaturationLimit=inf  LowerSaturationLimit=-inf  LinearizeAsGain=off  AntiWindupMode=none  Kb=1  TrackingMode=off  Kt=1  PParamMin=[]  PParamMax=[]  IParamMin=[]  IParamMax=[]  DParamMin=[]  DParamMax=[]  NParamMin=[]  NParamMax=[]  KbParamMin=[]  KbParamMax=[]  KtParamMin=[]  KtParamMax=[]  POutMin=[]  POutMax=[]  IOutMin=[]  IOutMax=[]  DOutMin=[]  DOutMax=[]  NOutMin=[]  NOutMax=[]  KbOutMin=[]  KbOutMax=[]  KtOutMin=[]  KtOutMax=[]  IntegratorOutMin=[]  IntegratorOutMax=[]  FilterOutMin=[]  FilterOutMax=[]  SumOutMin=[]  SumOutMax=[]  SumI1OutMin=[]  SumI1OutMax=[]  SumI2OutMin=[]  SumI2OutMax=[]  SumI3OutMin=[]  SumI3OutMax=[]  SumDOutMin=[]  SumDOutMax=[]  SaturationOutMin=[]  SaturationOutMax=[]  IntegratorContinuousStateAttributes=''  IntegratorStateMustResolveToSignalObject=off  IntegratorRTWStateStorageClass=Auto  FilterContinuousStateAttributes=''  FilterStateMustResolveToSignalObject=off  FilterRTWStateStorageClass=Auto  DifferentiatorICPrevScaledInput=0  DifferentiatorOutMin=[]  DifferentiatorOutMax=[]  FilterDiffOutCoefMin=[]  FilterDiffOutCoefMax=[]  SumDenOutMin=[]  SumDenOutMax=[]  SumNumOutMin=[]  SumNumOutMax=[]  ReciprocalOutMin=[]  ReciprocalOutMax=[]  DivideOutMin=[]  DivideOutMax=[]  TunerSelectOption=Transfer Function Based (PID Tuner App)
  emi_656 : Outport
  wires:
  emi_655/1 -> cfblk4/1
  cfblk4/1 -> emi_656/1

== system sampleModel7126_pp_1_1/cfblk278/cfblk15/cfblk6 ==
  emi_467 : Inport
  Action Port : ActionPort  ActionType=then
  cfblk6 : DiscreteZeroPole  Poles=[0 0.5]  Gain=1  SampleTime=-1
  emi_468 : Outport
  wires:
  emi_467/1 -> cfblk6/1
  cfblk6/1 -> emi_468/1

== system sampleModel7126_pp_1_1/cfblk278/cfblk15/emi_469 ==
  Action Port : ActionPort  ActionType=else
  emi_470 : Assertion

== system sampleModel7126_pp_1_1/cfblk278/cfblk15/emi_657 ==
  Action Port : ActionPort  ActionType=else
  emi_658 : Assertion

== system sampleModel7126_pp_1_1/cfblk280/cfblk13/cfblk7 ==
  emi_2006 : Inport
  emi_2007 : Inport  Port=2
  Action Port : ActionPort  ActionType=then
  cfblk7 : Delay  ShowEnablePort=on
      settings: InputPortMap=u0,e6
  emi_2008 : Outport
  wires:
  emi_2006/1 -> cfblk7/1
  emi_2007/1 -> cfblk7/2
  cfblk7/1 -> emi_2008/1

== system sampleModel7126_pp_1_1/cfblk280/cfblk13/emi_2009 ==
  Action Port : ActionPort  ActionType=else
  emi_2010 : Assertion

== system sampleModel7126_pp_1_1/cfblk284/cfblk10/cfblk3 ==
  emi_1376 : Inport
  Action Port : ActionPort  ActionType=then
  cfblk3 : Delay
  emi_1377 : Outport
  wires:
  emi_1376/1 -> cfblk3/1
  cfblk3/1 -> emi_1377/1

== system sampleModel7126_pp_1_1/cfblk284/cfblk10/cfblk6 ==
  emi_598 : Inport
  Action Port : ActionPort  ActionType=then
  cfblk6 : UnitDelay  SampleTime=-1
  emi_599 : Outport
  wires:
  emi_598/1 -> cfblk6/1
  cfblk6/1 -> emi_599/1

== system sampleModel7126_pp_1_1/cfblk284/cfblk10/emi_1378 ==
  Action Port : ActionPort  ActionType=else
  emi_1379 : Assertion
